simulink model "Airframe"  (R2023b)
settings: Solver=VariableStepAuto  StartTime=0.0  StopTime=10.0  RelTol=1e-3
values from neighbouring files (symbols this model uses):
  G_act = ss(A_act, B_act, C_act, D_act)    [main.m]    (also in main_dict.m; troubleshooting.m)
  G_m = ss(A_sp, B_sp, C_sp, D_sp)    [main.m]    (also in main_dict.m; troubleshooting.m)
settings Model: Creator=PierluigiMeneses  LastModifiedBy=PierluigiMeneses

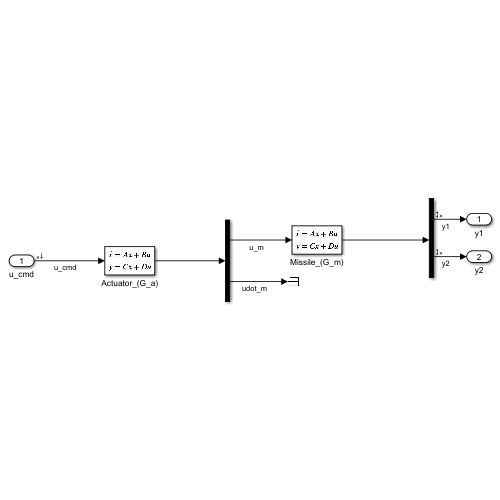
[thumbnail: Simulink's stored preview of the top-level diagram]
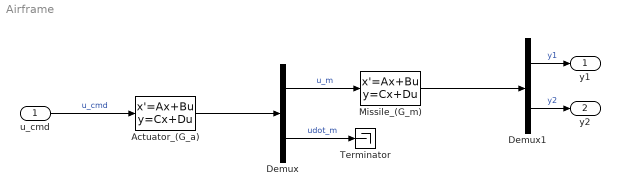
== system Airframe ==
  u_cmd : Inport
  Actuator_(G_a) : StateSpace  A=G_act.A  B=G_act.B  C=G_act.C  D=G_act.D  InitialCondition=0  ParameterTunability=Unconstrained
  Demux : Demux  Outputs=2
  Demux1 : Demux  Outputs=2
  Missile_(G_m) : StateSpace  A=G_m.A  B=G_m.B  C=G_m.C  D=G_m.D  InitialCondition=0
  Terminator : Terminator
  y1 : Outport
  y2 : Outport  Port=2
  wires:
  Actuator_(G_a)/1 -> Demux/1
  u_cmd/1 -> Actuator_(G_a)/1  "u_cmd"
  Demux/1 -> Missile_(G_m)/1  "u_m"
  Missile_(G_m)/1 -> Demux1/1
  Demux/2 -> Terminator/1  "udot_m"
  Demux1/1 -> y1/1  "y1"
  Demux1/2 -> y2/1  "y2"
